simulink model "CEGR_TestBench_10kW_SimplifiedEGR_v01_before_core_fix"  (R2025b)
settings: Solver=ode4  StartTime=0.0  StopTime=120  FixedStep=0.1  RelTol=1e-3
undefined symbols (not defined in the file): BenchBoundaryParam_simplified, EGRInitialNode_simplified, EgrSplitParam_simplified, I_stack_cmd_A_simplified, StackInitialState_simplified, StackParam_simplified
settings Model: Creator=ADMIN  LastModifiedBy=ADMIN

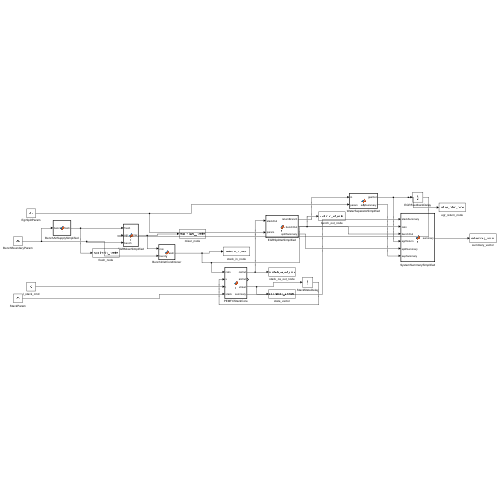
[thumbnail: Simulink's stored preview of the top-level diagram]
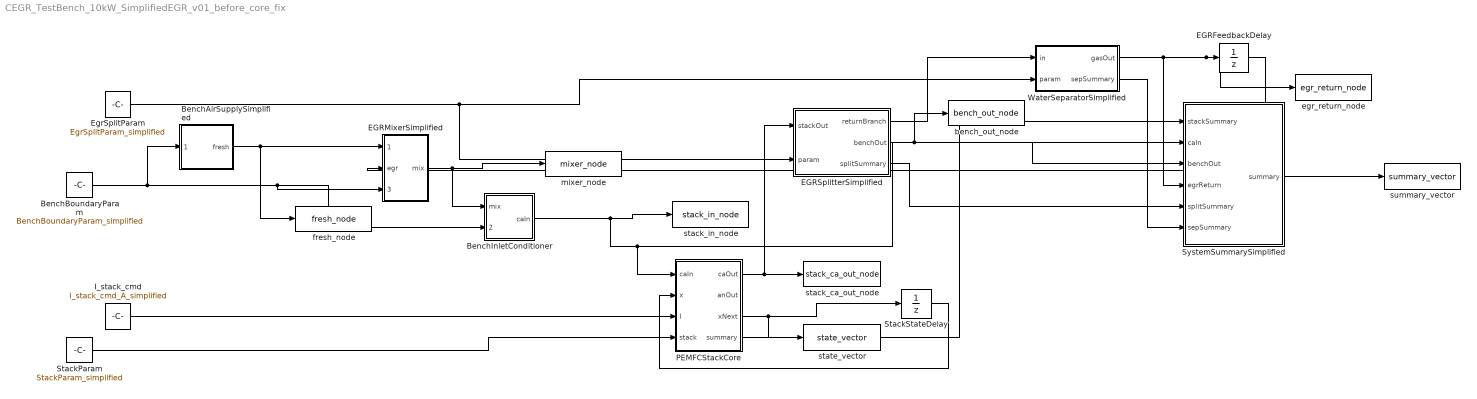
== system CEGR_TestBench_10kW_SimplifiedEGR_v01_before_core_fix ==
  BenchAirSupplySimplified : MATLAB Function  TreatAsAtomicUnit=on
  BenchBoundaryParam : Constant  Value=BenchBoundaryParam_simplified
  BenchInletConditioner : MATLAB Function  TreatAsAtomicUnit=on
  EGRFeedbackDelay : UnitDelay  InitialCondition=EGRInitialNode_simplified
  EGRMixerSimplified : MATLAB Function  TreatAsAtomicUnit=on
  EGRSplitterSimplified : MATLAB Function  TreatAsAtomicUnit=on
  EgrSplitParam : Constant  Value=EgrSplitParam_simplified
  I_stack_cmd : Constant  Value=I_stack_cmd_A_simplified
  PEMFCStackCore : MATLAB Function  TreatAsAtomicUnit=on
  StackParam : Constant  Value=StackParam_simplified
  StackStateDelay : UnitDelay  InitialCondition=StackInitialState_simplified
  SystemSummarySimplified : MATLAB Function  TreatAsAtomicUnit=on
  WaterSeparatorSimplified : MATLAB Function  TreatAsAtomicUnit=on
  bench_out_node : ToWorkspace  VariableName=bench_out_node  SaveFormat=Structure With Time
  egr_return_node : ToWorkspace  VariableName=egr_return_node  SaveFormat=Structure With Time
  fresh_node : ToWorkspace  VariableName=fresh_node  SaveFormat=Structure With Time
  mixer_node : ToWorkspace  VariableName=mixer_node  SaveFormat=Structure With Time
  stack_ca_out_node : ToWorkspace  VariableName=stack_ca_out_node  SaveFormat=Structure With Time
  stack_in_node : ToWorkspace  VariableName=stack_in_node  SaveFormat=Structure With Time
  state_vector : ToWorkspace  VariableName=state_vector  SaveFormat=Structure With Time
  summary_vector : ToWorkspace  VariableName=summary_vector  SaveFormat=Structure With Time
  wires:
  BenchBoundaryParam/1 -> BenchInletConditioner/2(bench), EGRMixerSimplified/3(bench), BenchAirSupplySimplified/1(bench)
  EgrSplitParam/1 -> WaterSeparatorSimplified/2(param), EGRSplitterSimplified/2(param)
  StackParam/1 -> PEMFCStackCore/4(stack)
  I_stack_cmd/1 -> PEMFCStackCore/3(I)
  StackStateDelay/1 -> PEMFCStackCore/2(x)
  BenchAirSupplySimplified/1(fresh) -> fresh_node/1, EGRMixerSimplified/1(fresh)
  EGRFeedbackDelay/1 -> EGRMixerSimplified/2(egr)
  EGRMixerSimplified/1(mix) -> mixer_node/1, BenchInletConditioner/1(mix)
  BenchInletConditioner/1(caIn) -> SystemSummarySimplified/2(caIn), PEMFCStackCore/1(caIn), stack_in_node/1
  PEMFCStackCore/1(caOut) -> EGRSplitterSimplified/1(stackOut), stack_ca_out_node/1
  WaterSeparatorSimplified/1(gasOut) -> SystemSummarySimplified/4(egrReturn), EGRFeedbackDelay/1, egr_return_node/1
  PEMFCStackCore/3(xNext) -> state_vector/1, StackStateDelay/1
  PEMFCStackCore/4(summary) -> SystemSummarySimplified/1(stackSummary)
  EGRSplitterSimplified/2(benchOut) -> bench_out_node/1, SystemSummarySimplified/3(benchOut)
  EGRSplitterSimplified/3(splitSummary) -> SystemSummarySimplified/5(splitSummary)
  WaterSeparatorSimplified/2(sepSummary) -> SystemSummarySimplified/6(sepSummary)
  SystemSummarySimplified/1(summary) -> summary_vector/1
  EGRSplitterSimplified/1(returnBranch) -> WaterSeparatorSimplified/1(in)

== matlab function CEGR_TestBench_10kW_SimplifiedEGR_v01_before_core_fix/EGRMixerSimplified ==
  data: fresh input; mix output; egr input; bench input
function mix = f(fresh, egr, bench)
%#codegen
mTarget=max(bench(9),1e-12); me0=max(sum(egr(1:3)),0); me=min(me0,0.95*mTarget); mf=max(mTarget-me,0);
wf=fresh(1:4)/max(sum(fresh(1:4)),1e-12); we=egr(1:4)/max(sum(egr(1:4)),1e-12);
mix=zeros(7,1); mix(1:4)=mf*wf+me*we; mt=max(mf+me,1e-12);
mix(5)=(fresh(5)*mf+egr(5)*me)/mt; mix(6)=fresh(6); mix(7)=double(mix(4)>1e-12);
end

== matlab function CEGR_TestBench_10kW_SimplifiedEGR_v01_before_core_fix/BenchAirSupplySimplified ==
  data: bench input; fresh output
function fresh = f(bench)
%#codegen
M_O2=bench(1); M_N2=bench(2); M_H2O=bench(3); p=bench(4); T=bench(5); RH=bench(6); xO2=bench(7); xN2=bench(8); mTarget=max(bench(10),1e-12);
pH2O=min(max(RH,0)*sat_kPa(T),0.98*p); yH2O=min(max(pH2O/max(p,1e-6),0),0.98);
yO2=(1-yH2O)*xO2; yN2=(1-yH2O)*xN2; mO2=yO2*M_O2; mN2=yN2*M_N2; mV=yH2O*M_H2O; s=max(mO2+mN2+mV,1e-12);
fresh=[mTarget*mO2/s; mTarget*mN2/s; mTarget*mV/s; 0; T; p; 0];
end
function p=sat_kPa(T)
Tc=min(max(T,-40),120); p=0.61121*exp((18.678-Tc/234.5)*(Tc/(257.14+Tc)));
end

== matlab function CEGR_TestBench_10kW_SimplifiedEGR_v01_before_core_fix/BenchInletConditioner ==
  data: mix input; caIn output; bench input
function caIn = f(mix, bench)
%#codegen
M_O2=bench(1); M_N2=bench(2); M_H2O=bench(3); p=bench(4); T=bench(5);
caIn=mix; caIn(5)=T; caIn(6)=p;
ps=min(sat_kPa(T),0.98*p); nDry=max(caIn(1)/M_O2+caIn(2)/M_N2,1e-12); mSat=ps*nDry/max(p-ps,1e-6)*M_H2O;
if caIn(3)>mSat, caIn(4)=caIn(4)+caIn(3)-mSat; caIn(3)=mSat; end
caIn(7)=double(caIn(4)>1e-12);
end
function p=sat_kPa(T)
Tc=min(max(T,-40),120); p=0.61121*exp((18.678-Tc/234.5)*(Tc/(257.14+Tc)));
end

== matlab function CEGR_TestBench_10kW_SimplifiedEGR_v01_before_core_fix/PEMFCStackCore ==
  data: caIn input; caOut output; x input; I input; stack input; anOut output; xNext output; summary output
function [caOut, anOut, xNext, summary] = f(caIn, x, I, stack)
%#codegen
% pcBack is the cathode outlet back-pressure boundary, not a predicted downstream pressure.
R=stack(1); F=stack(2); M_O2=stack(3); M_N2=stack(4); M_H2O=stack(5); M_H2=stack(6); pamb=stack(7); Tamb=stack(8); N=stack(9); A=stack(10);
Vca=stack(11); Van=stack(12); Kca=stack(13); Kan=stack(14); pcBack=stack(15); panBack=stack(16); Cfc=stack(18); hCool=stack(19); Tcool=stack(20); hAmb=stack(21);
Eref=stack(22); Etemp=stack(23); th1=stack(24); th2=stack(25); th3=stack(26); th4=stack(27); deltaCm=stack(28); th8=stack(29); th9=stack(30); th10=stack(31); Vtn=stack(32); anStoich=stack(33); RHAn=stack(34); dt=stack(35); panIn=stack(37); KcaIn=stack(38); th5=stack(72); th6=stack(73); th7=stack(74); egrFrac=0; egrLossK=0; egrLossExp=1; egrLossRh=0; if numel(stack)>=78, egrFrac=stack(75); egrLossK=stack(76); egrLossExp=max(stack(77),0.2); egrLossRh=stack(78); end
coolantFlow=stack(44);
hCoolEff=hCool; if numel(stack)>=71 && stack(45)>0.5, hCoolEff=interp_hcool_flow(coolantFlow,stack(46:58),stack(59:71),hCool); end
mO2=max(x(1),1e-12); mN2=max(x(2),1e-12); mV=max(x(3),0); mH2=max(x(4),1e-12); mVAn=max(x(5),0); T=x(6); TK=T+273.15;
pO2=mO2/M_O2*R*TK/Vca/1000; pN2=mN2/M_N2*R*TK/Vca/1000; pV=mV/M_H2O*R*TK/Vca/1000; pCa=max(pO2+pN2+pV,pamb);
pVAn=mVAn/M_H2O*R*TK/Van/1000;
mInCmd=sum(caIn(1:3)); mInPressure=KcaIn*max(caIn(6)-pCa,0); mIn=min(mInCmd,mInPressure); wIn=caIn(1:3)/max(mInCmd,1e-12); mO2In=mIn*wIn(1); mN2In=mIn*wIn(2); mVIn=mIn*wIn(3);
mO2React=I*N/(4*F)*M_O2; mH2React=I*N/(2*F)*M_H2; mWater=I*N/(2*F)*M_H2O; lambdaO2=(mO2In/M_O2)/max(I*N/(4*F),1e-12);
ps=sat_kPa(T); aCa=min(max(pV/max(ps,1e-6),0),3); aAn=min(max(pVAn/max(ps,1e-6),0),3); lam=0.5*(lambda_eq(aCa)+lambda_eq(aAn));
A_m2=A*1e-4; nDrag=max(0.0029*lam^2+0.05*lam,0); D=membrane_diff(lam,TK); cCa=pV*1000/(R*TK); cAn=pVAn*1000/(R*TK); mMem=(nDrag*I/F - D*A_m2*N/max(deltaCm*0.01,1e-9)*(cCa-cAn))*M_H2O;
mH2In=anStoich*mH2React; pH2OIn=RHAn*ps; mVAnIn=mH2In*max(pH2OIn,0)/max(panIn-pH2OIn,1e-6)*(M_H2O/M_H2);
mO2Pre=max(mO2+dt*(mO2In-mO2React),1e-12); mN2Pre=max(mN2+dt*mN2In,1e-12); mVPre=max(mV+dt*(mVIn+mWater+mMem),0);
mH2Pre=max(mH2+dt*(mH2In-mH2React),1e-12); mVAnPre=max(mVAn+dt*(mVAnIn-mMem),0);
pO2Pre=mO2Pre/M_O2*R*TK/Vca/1000; pN2Pre=mN2Pre/M_N2*R*TK/Vca/1000; pVPre=mVPre/M_H2O*R*TK/Vca/1000; pCaPre=max(pO2Pre+pN2Pre+pVPre,pamb);
pH2Pre=mH2Pre/M_H2*R*TK/Van/1000; pVAnPre=mVAnPre/M_H2O*R*TK/Van/1000; pAnPre=max(pH2Pre+pVAnPre,pamb);
gasCa=max(mO2Pre+mN2Pre+mVPre,1e-12); wO2=mO2Pre/gasCa; wN2=mN2Pre/gasCa; wV=mVPre/gasCa;
mCaOutRaw=Kca*max(pCaPre-pcBack,0)/(1+Kca*max(pCaPre,1e-6)*dt/gasCa); mCaOut=min(mCaOutRaw,0.95*gasCa/max(dt,1e-9));
gasAn=max(mH2Pre+mVAnPre,1e-12); wH2=mH2Pre/gasAn; wVAn=mVAnPre/gasAn;
mAnOutRaw=Kan*max(pAnPre-panBack,0)/(1+Kan*max(pAnPre,1e-6)*dt/gasAn); mAnOut=min(mAnOutRaw,0.95*gasAn/max(dt,1e-9));
mO2n=max(mO2Pre-dt*wO2*mCaOut,1e-12); mN2n=max(mN2Pre-dt*wN2*mCaOut,1e-12); mVnRaw=max(mVPre-dt*wV*mCaOut,0);
mH2n=max(mH2Pre-dt*wH2*mAnOut,1e-12); mVAnnRaw=max(mVAnPre-dt*wVAn*mAnOut,0);
[mVn,liqDiag]=clip_vapor(mVnRaw,0,mO2n,mN2n,T,pCaPre,stack,0); [mVAnn,liqAnDiag]=clip_vapor(mVAnnRaw,0,mH2n,0,T,pAnPre,stack,1);
phaseCa=(mVnRaw-mVn)/dt; phaseAn=(mVAnnRaw-mVAnn)/dt;
j=max(I/max(A,1e-9),1e-6); E=Eref-Etemp*(TK-298.15)+R*TK/(2*F)*log(max(pH2Pre*1000,1)/101325*sqrt(max(pO2Pre*1000,1)/101325));
CO2=max(1.97e-7*(pO2Pre*1000)*exp(498/TK),1e-12); etaAct=max(th1+th2*TK+th3*TK*log(CO2)+th4*TK*log(max(I,1e-6)),0);
Rm=deltaCm/max(A*(th5*lam+th6)*exp(th7*(1/303.15-1/TK)),1e-12); etaOhm=I*(Rm+th8);
iLim=j; i0Scale=CO2; etaCon=max(th9*exp(min(th10*I,50)),0); egrLoss=max(egrLossK,0)*max(egrFrac,0)^egrLossExp + max(egrLossRh,0)*max(aCa-0.8,0)*max(egrFrac,0); etaCon=etaCon+max(egrLoss,0);
V=E-etaAct-etaOhm-etaCon; Pstack=I*V*N; Qgen=I*N*(Vtn-V); Qcool=hCoolEff*(T-Tcool); Qamb=hAmb*(T-Tamb); Qgas=max(mCaOut+mAnOut,0)*1050*max(T-caIn(5),0); Qnet=Qgen-Qcool-Qamb-Qgas; Tn=T+dt*Qnet/Cfc;
TKn=Tn+273.15; pO2Diag=mO2n/M_O2*R*TKn/Vca/1000; pN2Diag=mN2n/M_N2*R*TKn/Vca/1000; pVDiag=mVn/M_H2O*R*TKn/Vca/1000; pCaDiag=max(pO2Diag+pN2Diag+pVDiag,pamb);
pH2Diag=mH2n/M_H2*R*TKn/Van/1000; pVAnDiag=mVAnn/M_H2O*R*TKn/Van/1000; pAnDiag=max(pH2Diag+pVAnDiag,pamb);
xNext=[mO2n;mN2n;mVn;mH2n;mVAnn;Tn]; caOut=[wO2*mCaOut;wN2*mCaOut;wV*mCaOut;0;Tn+3;pcBack;0]; anOut=[wH2*mAnOut;0;wVAn*mAnOut;0;Tn;panBack;0];
nTot=max(mO2n/M_O2+mN2n/M_N2+mVn/M_H2O,1e-12); xO2=(mO2n/M_O2)/nTot; RH=(mVn/M_H2O*R*(Tn+273.15)/Vca/1000)/max(sat_kPa(Tn),1e-6);
nInTot=max(caIn(1)/M_O2+caIn(2)/M_N2+caIn(3)/M_H2O,1e-12); xO2In=(caIn(1)/M_O2)/nInTot; pO2In=caIn(6)*xO2In; RHIn=(caIn(6)*(caIn(3)/M_H2O)/nInTot)/max(sat_kPa(caIn(5)),1e-6);
resO2=(mO2n-mO2)/dt-(mO2In-wO2*mCaOut-mO2React); resN2=(mN2n-mN2)/dt-(mN2In-wN2*mCaOut);
resH2Ov=(mVn-mV)/dt-(mVIn-wV*mCaOut+mWater+mMem-phaseCa);
resH2=(mH2n-mH2)/dt-(mH2In-wH2*mAnOut-mH2React); resH2OvAn=(mVAnn-mVAn)/dt-(mVAnIn-wVAn*mAnOut-mMem-phaseAn);
maxGasRes=max(abs([resO2,resN2,resH2Ov,resH2,resH2OvAn]));
summary=[I;V;Pstack;pO2Diag;pCaDiag;pH2Diag;pAnDiag;lam;Tn;xO2;RH;mMem;mO2React;mH2React;mWater;mCaOut;mAnOut;Cfc*(Tn-T)/dt-Qnet;pO2In;xO2In;RHIn;Qnet;resO2;resN2;resH2Ov;phaseCa;resH2;resH2OvAn;phaseAn;phaseCa+phaseAn;maxGasRes;Qgen;Qcool;Qamb;Qgas;E;etaAct;etaOhm;etaCon;lambdaO2;mIn;iLim;i0Scale;mVIn;wV*mCaOut;mVAnIn;wVAn*mAnOut;liqDiag+liqAnDiag];
end
function [mv,ml]=clip_vapor(mv0,ml0,mA,mB,T,p,stack,isAnode)
M_O2=stack(3); M_N2=stack(4); M_H2O=stack(5); M_H2=stack(6); MA=M_O2; MB=M_N2; if isAnode>0.5, MA=M_H2; end; ps=min(sat_kPa(T),0.98*p); nDry=max(mA/MA+mB/MB,1e-12); mSat=max(ps*nDry/max(p-ps,1e-6)*M_H2O,0); if mv0>mSat, mv=mSat; ml=ml0+mv0-mSat; else, mv=mv0; ml=ml0; end
end
function p=sat_kPa(T)
Tc=min(max(T,-40),120); p=0.61121*exp((18.678-Tc/234.5)*(Tc/(257.14+Tc)));
end
function lambda=lambda_eq(a)
if a<=1, lambda=0.043+17.81*a-39.85*a^2+36*a^3; else, lambda=14+1.4*(a-1); end
end
function D=membrane_diff(lambda,TK)
if lambda<2, d0=1e-10; elseif lambda<3, d0=1e-10*(1+2*(lambda-2)); elseif lambda<4.5, d0=1e-10*(3-1.167*(lambda-3)); else, d0=1.25e-10; end; D=d0*exp(2416*(1/303-1/max(TK,1)));
end
function h=interp_hcool_flow(flow,bp,hv,hFallback)
n=0; for k=1:numel(bp), if bp(k)>0 && hv(k)>0, n=n+1; end, end; if n<2, h=hFallback; return; end
b=zeros(n,1); v=zeros(n,1); j=0; for k=1:numel(bp), if bp(k)>0 && hv(k)>0, j=j+1; b(j)=bp(k); v(j)=hv(k); end, end
if flow<=b(1), h=v(1); return; end; if flow>=b(n), h=v(n); return; end
h=v(n); for k=1:n-1, if flow>=b(k) && flow<=b(k+1), a=(flow-b(k))/max(b(k+1)-b(k),1e-9); h=v(k)+a*(v(k+1)-v(k)); return; end, end
end

== matlab function CEGR_TestBench_10kW_SimplifiedEGR_v01_before_core_fix/EGRSplitterSimplified ==
  data: stackOut input; returnBranch output; param input; benchOut output; splitSummary output
function [returnBranch, benchOut, splitSummary] = f(stackOut, param)
%#codegen
r=min(max(param(1),0),0.95); returnBranch=stackOut; returnBranch(1:4)=r*stackOut(1:4); returnBranch(7)=double(returnBranch(4)>1e-12);
benchOut=stackOut; benchOut(1:4)=(1-r)*stackOut(1:4); benchOut(7)=double(benchOut(4)>1e-12);
mOutGas=sum(stackOut(1:3)); splitSummary=[r;sum(returnBranch(1:3));sum(benchOut(1:3));mOutGas;stackOut(4);returnBranch(4);benchOut(4);param(4);param(5)];
end

== matlab function CEGR_TestBench_10kW_SimplifiedEGR_v01_before_core_fix/WaterSeparatorSimplified ==
  data: in input; gasOut output; param input; sepSummary output
function [gasOut, sepSummary] = f(in, param)
%#codegen
M_O2=0.031998; M_N2=0.0280134; M_H2O=0.01801528; gasOut=in; gasOut(5)=param(2); gasOut(6)=param(3);
p=max(gasOut(6),1e-6); T=gasOut(5); ps=min(sat_kPa(T),0.98*p); nDry=max(gasOut(1)/M_O2+gasOut(2)/M_N2,1e-12); mSat=ps*nDry/max(p-ps,1e-6)*M_H2O;
condensed=max(gasOut(3)-mSat,0); gasOut(3)=gasOut(3)-condensed; drain=gasOut(4)+condensed; gasOut(4)=0; gasOut(7)=0;
sepSummary=[drain;condensed;in(4);rel_hum(gasOut,M_O2,M_N2,M_H2O);T;p;sum(gasOut(1:3))];
end
function rh=rel_hum(node,M_O2,M_N2,M_H2O)
nV=max(node(3)/M_H2O,0); nt=max(node(1)/M_O2+node(2)/M_N2+nV,1e-12); rh=node(6)*nV/nt/max(sat_kPa(node(5)),1e-6);
end
function p=sat_kPa(T)
Tc=min(max(T,-40),120); p=0.61121*exp((18.678-Tc/234.5)*(Tc/(257.14+Tc)));
end

== matlab function CEGR_TestBench_10kW_SimplifiedEGR_v01_before_core_fix/SystemSummarySimplified ==
  data: stackSummary input; summary output; caIn input; benchOut input; egrReturn input; splitSummary input; sepSummary input
function summary = f(stackSummary, caIn, benchOut, egrReturn, splitSummary, sepSummary)
%#codegen
M_O2=0.031998; M_N2=0.0280134; M_H2O=0.01801528; nIn=max(caIn(1)/M_O2+caIn(2)/M_N2+caIn(3)/M_H2O,1e-12);
xO2In=(caIn(1)/M_O2)/nIn; mIn=sum(caIn(1:3)); mEgr=sum(egrReturn(1:3)); mBenchOut=sum(benchOut(1:3));
summary=[stackSummary; xO2In; mIn; mEgr; mBenchOut; splitSummary; sepSummary];
end
